simulink model "SB_SC_AM_system"  (R2021a)
settings: Solver=VariableStepAuto  StartTime=0.0  StopTime=10.0  RelTol=1e-3
settings Model: Creator=Fatiha  LastModifiedBy=Fatiha

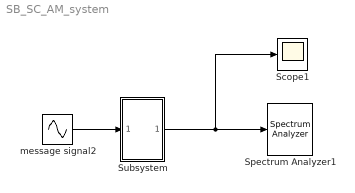
== system SB_SC_AM_system ==
  Scope1 : Scope
  Spectrum Analyzer1 : SpectrumAnalyzer
  Subsystem : Subsystem
  message signal2 : Sin  Frequency=2*pi*50  Phase=pi/2  SampleTime=0.00001
  wires:
  message signal2/1 -> Subsystem/1(In1)
  Subsystem/1(Out1) -> Spectrum Analyzer1/1, Scope1/1

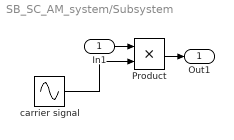
== system SB_SC_AM_system/Subsystem ==
  In1 : Inport
  Product : Product
  carrier signal : Sin  Frequency=2*pi*1000  Phase=pi/2  SampleTime=0.00001
  Out1 : Outport
  wires:
  carrier signal/1 -> Product/2
  Product/1 -> Out1/1
  In1/1 -> Product/1
